simulink model "Qn7"  (R2022b)
settings: Solver=VariableStepAuto  StartTime=0.0  StopTime=10.0  MaxStep=0.01  RelTol=1e-3
settings Model: Creator=nmary  LastModifiedBy=nmary

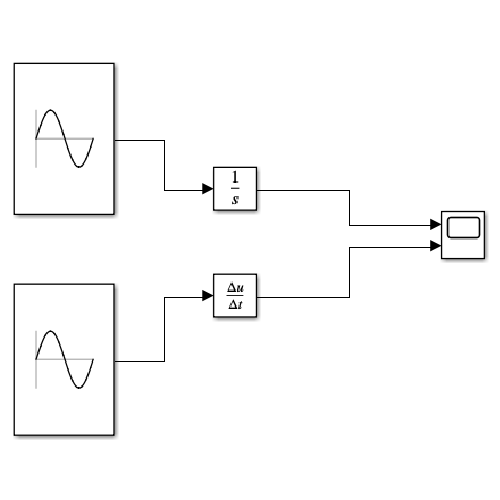
[thumbnail: Simulink's stored preview of the top-level diagram]
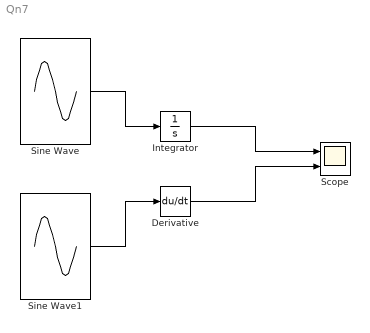
== system Qn7 ==
  Derivative : Derivative
  Integrator : Integrator  InitialCondition=-1
  Scope : Scope  NumInputPorts=2
  Sine Wave : Sin  SampleTime=0
  Sine Wave1 : Sin  SampleTime=0
  wires:
  Sine Wave/1 -> Integrator/1
  Integrator/1 -> Scope/1
  Sine Wave1/1 -> Derivative/1
  Derivative/1 -> Scope/2
